simulink model "PlantWithDelayTest"  (R2017a)
settings: Solver=FixedStepAuto  StartTime=0.0  StopTime=25  FixedStep=0.0025  RelTol=1e-3
undefined symbols (not defined in the file): alp, Standard_Devices, UDP_Protocol
libraries: sldrtlib x2
settings Model: Creator=wangy  LastModifiedBy=wangy

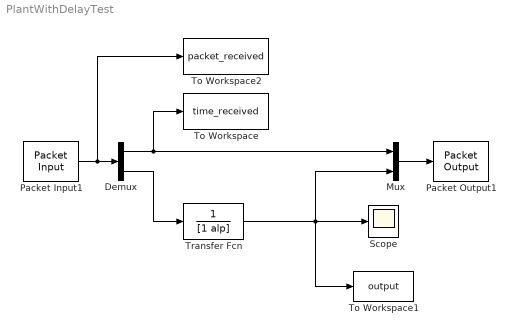
== system PlantWithDelayTest ==
  Demux : Demux  Outputs=2
  Mux : Mux  Inputs=2
  Packet Input1 : sldrtlib/Packet Input  Priority=0  SampleTime=0.01  MaxMissedTicks=inf  ShowMissedTicks=off  YieldWhenWaiting=off  DrvName=Standard_Devices/UDP_Protocol  DrvAddress=12002  DrvOptions=[425774274 12003]  PacketSize=16  DataTypes='2*double'  ShowReady=off  ShowError=off  PacketID=1  ByteOrder=1  ShowTimestamp=off
      settings: AttributesFormatString=Standard Devices\nUDP Protocol [2EE2h]  SourceProductName=Simulink Desktop Real-Time
  Packet Output1 : sldrtlib/Packet Output  Priority=2  SampleTime=0.01  MaxMissedTicks=inf  ShowMissedTicks=off  YieldWhenWaiting=off  DrvName=Standard_Devices/UDP_Protocol  DrvAddress=12000  DrvOptions=[425774274 12001]  PacketSize=16  DataTypes='2*double'  ShowReady=off  ShowError=off  PacketID=1  ByteOrder=1  InitialValue=[]  FinalValue=[]
      settings: AttributesFormatString=Standard Devices\nUDP Protocol [2EE0h]  SourceProductName=Simulink Desktop Real-Time
  Scope : Scope
  To Workspace : ToWorkspace  VariableName=time_received  SaveFormat=Timeseries  SampleTime=-1
  To Workspace1 : ToWorkspace  VariableName=output  SaveFormat=Timeseries  SampleTime=-1
  To Workspace2 : ToWorkspace  VariableName=packet_received  SaveFormat=Timeseries  SampleTime=-1
  Transfer Fcn : TransferFcn  Priority=1  Denominator=[1 alp]
  wires:
  Packet Input1/1 -> To Workspace2/1, Demux/1
  Demux/2 -> Transfer Fcn/1
  Demux/1 -> To Workspace/1, Mux/1
  Transfer Fcn/1 -> Mux/2, To Workspace1/1, Scope/1
  Mux/1 -> Packet Output1/1
